simulink model "Thermostat_PI_Controller"  (R2025a)
settings: Solver=VariableStepAuto  StartTime=0.0  StopTime=10.0  RelTol=1e-3
undefined symbols (not defined in the file): ki, kp, Ts, X

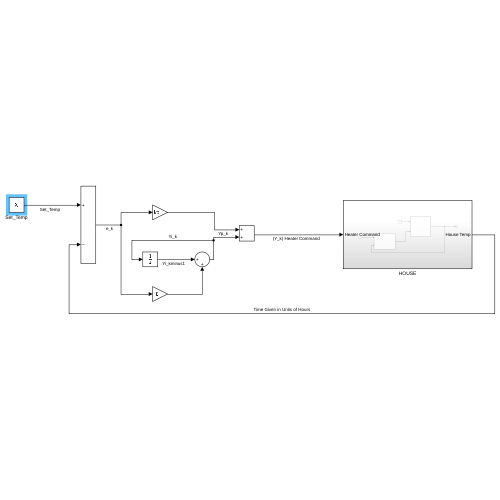
[thumbnail: Simulink's stored preview of the top-level diagram]
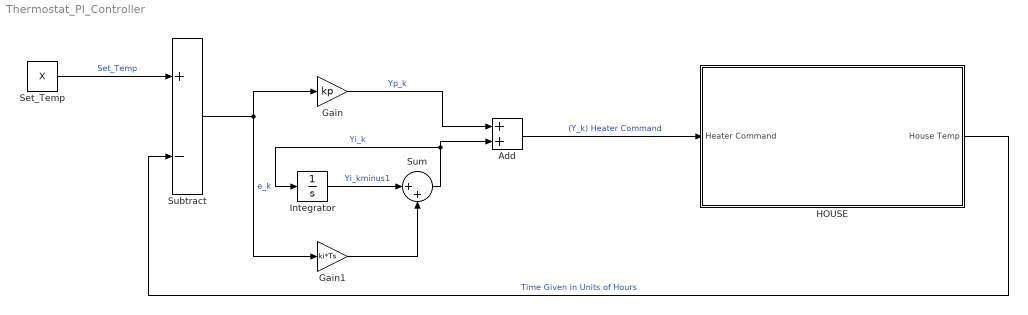
== system Thermostat_PI_Controller ==
  Add : Sum
  Gain : Gain  Gain=kp
  Gain1 : Gain  Gain=ki*Ts
  HOUSE : Subsystem
  Integrator : Integrator
  Set_Temp : Constant  Value=X
  Subtract : Sum  Inputs=+-
  Sum : Sum  Inputs=|++
  wires:
  Set_Temp/1 -> Subtract/1  "Set_Temp"
  Subtract/1 -> Gain/1, Gain1/1  "e_k"
  Gain/1 -> Add/1  "Yp_k"
  Add/1 -> HOUSE/1(Heater Command)  "(Y_k) Heater Command"
  Gain1/1 -> Sum/2
  Integrator/1 -> Sum/1  "Yi_kminus1"
  Sum/1 -> Add/2, Integrator/1  "Yi_k"
  HOUSE/1(House Temp) -> Subtract/2  "Time Given in Units of Hours"

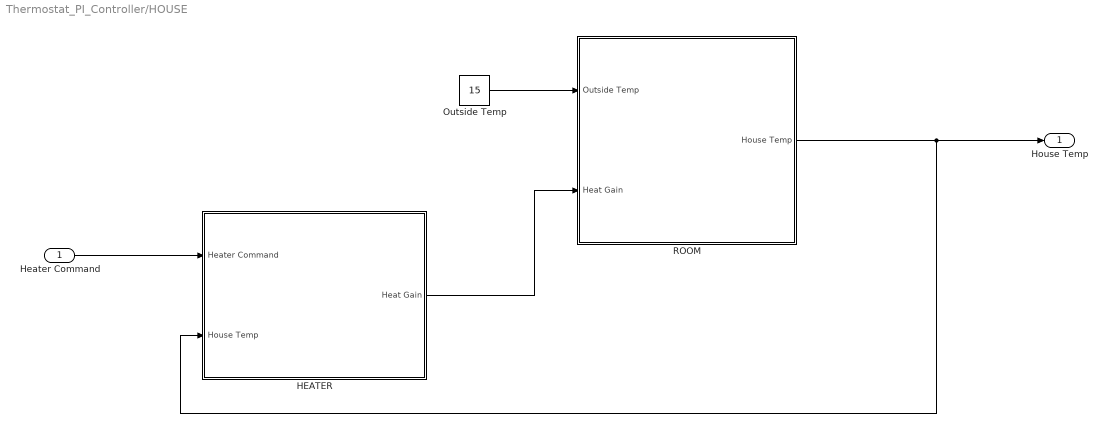
== system Thermostat_PI_Controller/HOUSE ==
  Heater Command : Inport
  HEATER : Subsystem
  Outside Temp : Constant  Value=15
  ROOM : Subsystem
  House Temp : Outport
  wires:
  Outside Temp/1 -> ROOM/1(Outside Temp)
  ROOM/1(House Temp) -> HEATER/2(House Temp), House Temp/1
  Heater Command/1 -> HEATER/1(Heater Command)
  HEATER/1(Heat Gain) -> ROOM/2(Heat Gain)

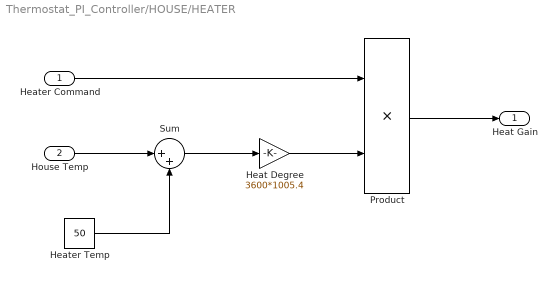
== system Thermostat_PI_Controller/HOUSE/HEATER ==
  Heater Command : Inport
  House Temp : Inport  Port=2
  Heat Degree : Gain  Gain=3600*1005.4
  Heater Temp : Constant  Value=50
  Product : Product
  Sum : Sum  Inputs=|++
  Heat Gain : Outport
  wires:
  House Temp/1 -> Sum/1
  Heater Command/1 -> Product/1
  Heat Degree/1 -> Product/2
  Product/1 -> Heat Gain/1
  Heater Temp/1 -> Sum/2
  Sum/1 -> Heat Degree/1

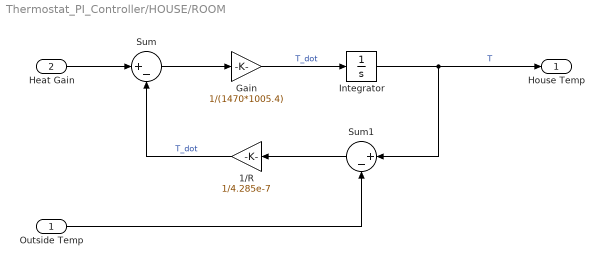
== system Thermostat_PI_Controller/HOUSE/ROOM ==
  Outside Temp : Inport
  Heat Gain : Inport  Port=2
  1/R : Gain  Gain=1/4.285e-7
  Gain : Gain  Gain=1/(1470*1005.4)
  Integrator : Integrator
  Sum : Sum  Inputs=|+-
  Sum1 : Sum  Inputs=|+-
  House Temp : Outport
  wires:
  Outside Temp/1 -> Sum1/2
  Heat Gain/1 -> Sum/1
  Gain/1 -> Integrator/1  "T_dot"
  Sum/1 -> Gain/1
  Sum1/1 -> 1/R/1
  1/R/1 -> Sum/2  "T_dot"
  Integrator/1 -> House Temp/1, Sum1/1  "T"
